simulink model "KE88_visualizacion"  (R2026a)
settings: Solver=VariableStepAuto
InitFcn:
  | KE88_parametros
undefined symbols (not defined in the file or in its folder): KE88_dibujo

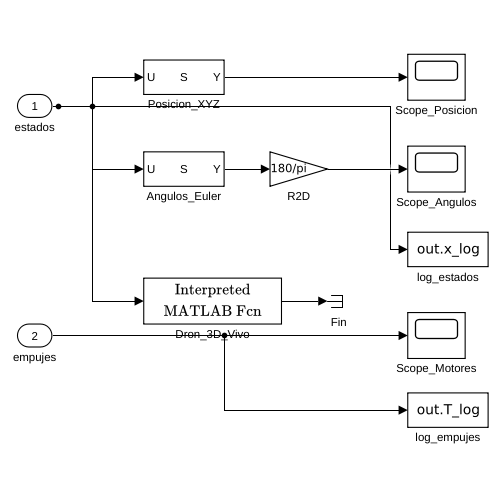
[thumbnail: Simulink's stored preview of the top-level diagram]
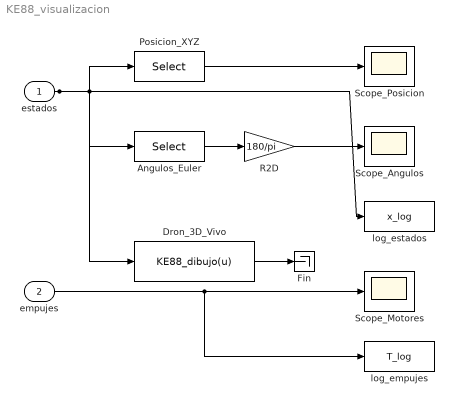
== system KE88_visualizacion ==
  estados : Inport  PortDimensions=12
  empujes : Inport  Port=2  PortDimensions=4
  Angulos_Euler : Selector  InputPortWidth=12  IndexOptions=Index vector (dialog)  Indices=[7 8 9]  OutputSizes=1
  Dron_3D_Vivo : MATLABFcn  MATLABFcn=KE88_dibujo(u)  OutputDimensions=1
  Fin : Terminator
  Posicion_XYZ : Selector  InputPortWidth=12  IndexOptions=Index vector (dialog)  Indices=[1 2 3]  OutputSizes=1
  R2D : Gain  Gain=180/pi
  Scope_Angulos : Scope
  Scope_Motores : Scope
  Scope_Posicion : Scope
      settings: ActiveDisplayYMinimum=-19.724253696422878  ActiveDisplayYMaximum=177.51828326780594
  log_empujes : ToWorkspace  VariableName=T_log  SaveFormat=Structure With Time  SampleTime=-1
  log_estados : ToWorkspace  VariableName=x_log  SaveFormat=Structure With Time  SampleTime=-1
  wires:
  estados/1 -> Posicion_XYZ/1, Angulos_Euler/1, log_estados/1, Dron_3D_Vivo/1
  Posicion_XYZ/1 -> Scope_Posicion/1
  Angulos_Euler/1 -> R2D/1
  R2D/1 -> Scope_Angulos/1
  empujes/1 -> Scope_Motores/1, log_empujes/1
  Dron_3D_Vivo/1 -> Fin/1
